simulink model "radix2_N128"  (R2024b)
settings: Solver=VariableStepAuto  StartTime=0.0  StopTime=1  RelTol=1e-3
settings Model: Creator=gjp88  LastModifiedBy=gjp88
settings SolverCC: AlgebraicLoopSolver=TrustRegion
settings DebuggingCC: UnconnectedInputMsg=warning  UnconnectedOutputMsg=warning  UnconnectedLineMsg=warning
settings ModelReferenceCC: EnableRefExpFcnMdlSchedulingChecks=on
settings RTWCC: GPUComputeCapability=3.5

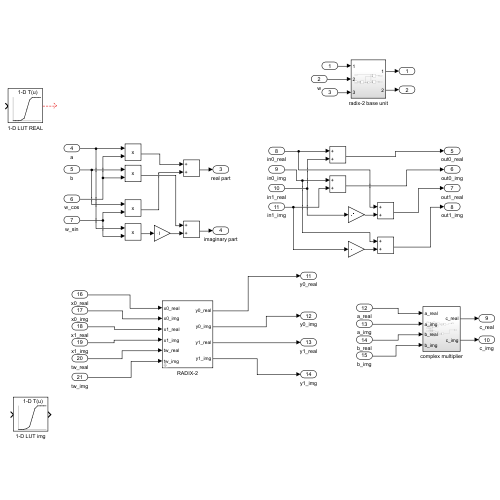
[thumbnail: Simulink's stored preview of the top-level diagram]
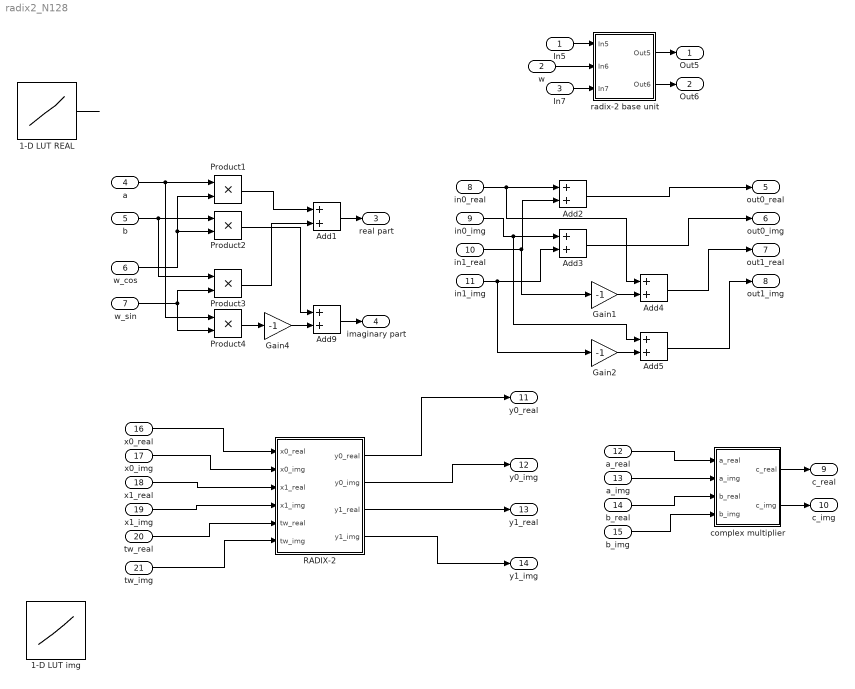
== system radix2_N128 ==
  In5 : Inport
  w : Inport  Port=2
  In7 : Inport  Port=3
  a : Inport  Port=4
  b : Inport  Port=5
  w_cos : Inport  Port=6
  w_sin : Inport  Port=7
  in0_real : Inport  Port=8
  in0_img : Inport  Port=9
  in1_real : Inport  Port=10
  in1_img : Inport  Port=11
  a_real : Inport  Port=12
  a_img : Inport  Port=13
  b_real : Inport  Port=14
  b_img : Inport  Port=15
  x0_real : Inport  Port=16
  x0_img : Inport  Port=17
  x1_real : Inport  Port=18
  x1_img : Inport  Port=19
  tw_real : Inport  Port=20
  tw_img : Inport  Port=21
  1-D LUT REAL : Lookup_n-D  NumberOfTableDimensions=1  BreakpointsForDimension1=[-5:5]  Table=tanh([-5:5])  InternalRulePriority=Speed  RndMeth=Simplest
  1-D LUT img : Lookup_n-D  NumberOfTableDimensions=1  BreakpointsForDimension1=[-5:5]  Table=tanh([-5:5])  InternalRulePriority=Speed  RndMeth=Simplest
  Add{1..5,9} (6 alike) : Sum
  Gain1 : Gain  Gain=-1
  Gain2 : Gain  Gain=-1
  Gain4 : Gain  Gain=-1
  Product{1..4} (4 alike) : Product
  RADIX-2 : Subsystem
      mask DialogControl RADIX_BUTTERFLY Prompt: RADIX-2
      mask DialogControl ParameterGroupVar Prompt: 参数
  complex multiplier : Subsystem
  radix-2 base unit : Subsystem
  Out5 : Outport
  Out6 : Outport  Port=2
  real part : Outport  Port=3
  imaginary part : Outport  Port=4
  out0_real : Outport  Port=5
  out0_img : Outport  Port=6
  out1_real : Outport  Port=7
  out1_img : Outport  Port=8
  c_real : Outport  Port=9
  c_img : Outport  Port=10
  y0_real : Outport  Port=11
  y0_img : Outport  Port=12
  y1_real : Outport  Port=13
  y1_img : Outport  Port=14
  wires:
  Gain4/1 -> Add9/2
  In5/1 -> radix-2 base unit/1(In5)
  a/1 -> Product4/1, Product1/1
  Product4/1 -> Gain4/1
  Add9/1 -> imaginary part/1
  Add1/1 -> real part/1
  Product1/1 -> Add1/1
  Product2/1 -> Add9/1
  Product3/1 -> Add1/2
  radix-2 base unit/2(Out6) -> Out6/1
  w_cos/1 -> Product2/2, Product1/2
  w/1 -> radix-2 base unit/2(In6)
  w_sin/1 -> Product3/2, Product4/2
  radix-2 base unit/1(Out5) -> Out5/1
  b/1 -> Product3/1, Product2/1
  In7/1 -> radix-2 base unit/3(In7)
  1-D LUT REAL/1 -> ?
  Gain1/1 -> Add4/2
  in0_real/1 -> Add4/1, Add2/1
  in1_real/1 -> Gain1/1, Add2/2
  Add4/1 -> out1_real/1
  Gain2/1 -> Add5/2
  in0_img/1 -> Add5/1, Add3/1
  in1_img/1 -> Gain2/1, Add3/2
  Add5/1 -> out1_img/1
  Add2/1 -> out0_real/1
  Add3/1 -> out0_img/1
  a_real/1 -> complex multiplier/1(a_real)
  a_img/1 -> complex multiplier/2(a_img)
  b_real/1 -> complex multiplier/3(b_real)
  b_img/1 -> complex multiplier/4(b_img)
  complex multiplier/1(c_real) -> c_real/1
  complex multiplier/2(c_img) -> c_img/1
  x0_real/1 -> RADIX-2/1(x0_real)
  x0_img/1 -> RADIX-2/2(x0_img)
  x1_real/1 -> RADIX-2/3(x1_real)
  x1_img/1 -> RADIX-2/4(x1_img)
  tw_real/1 -> RADIX-2/5(tw_real)
  tw_img/1 -> RADIX-2/6(tw_img)
  RADIX-2/1(y0_real) -> y0_real/1
  RADIX-2/2(y0_img) -> y0_img/1
  RADIX-2/3(y1_real) -> y1_real/1
  RADIX-2/4(y1_img) -> y1_img/1

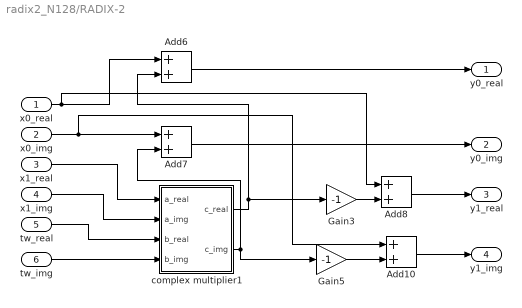
== system radix2_N128/RADIX-2 ==
  x0_real : Inport
  x0_img : Inport  Port=2
  x1_real : Inport  Port=3
  x1_img : Inport  Port=4
  tw_real : Inport  Port=5
  tw_img : Inport  Port=6
  Add{6..8,10} (4 alike) : Sum
  Gain3 : Gain  Gain=-1
  Gain5 : Gain  Gain=-1
  complex multiplier1 : Subsystem
  y0_real : Outport
  y0_img : Outport  Port=2
  y1_real : Outport  Port=3
  y1_img : Outport  Port=4
  wires:
  x0_img/1 -> Add10/1, Add7/1
  x1_real/1 -> complex multiplier1/1(a_real)
  Add10/1 -> y1_img/1
  tw_img/1 -> complex multiplier1/4(b_img)
  tw_real/1 -> complex multiplier1/3(b_real)
  Add7/1 -> y0_img/1
  Gain3/1 -> Add8/2
  x0_real/1 -> Add8/1, Add6/1
  Add6/1 -> y0_real/1
  complex multiplier1/2(c_img) -> Add7/2, Gain5/1
  Gain5/1 -> Add10/2
  complex multiplier1/1(c_real) -> Add6/2, Gain3/1
  x1_img/1 -> complex multiplier1/2(a_img)
  Add8/1 -> y1_real/1

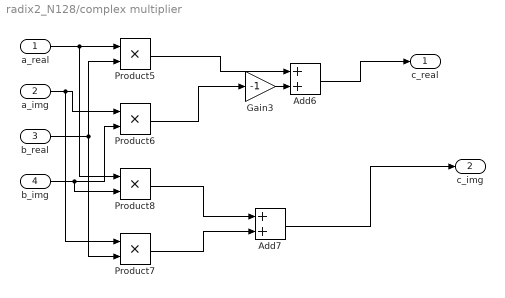
== system radix2_N128/complex multiplier ==
  a_real : Inport
  a_img : Inport  Port=2
  b_real : Inport  Port=3
  b_img : Inport  Port=4
  Add6 : Sum
  Add7 : Sum
  Gain3 : Gain  Gain=-1
  Product{5..8} (4 alike) : Product
  c_real : Outport
  c_img : Outport  Port=2
  wires:
  Product7/1 -> Add7/2
  Add6/1 -> c_real/1
  a_real/1 -> Product8/1, Product5/1
  Add7/1 -> c_img/1
  Product8/1 -> Add7/1
  Product5/1 -> Add6/1
  b_img/1 -> Product8/2, Product6/2
  a_img/1 -> Product7/1, Product6/1
  b_real/1 -> Product7/2, Product5/2
  Gain3/1 -> Add6/2
  Product6/1 -> Gain3/1

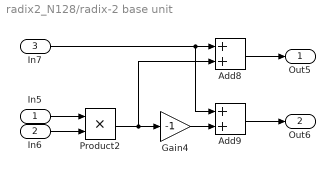
== system radix2_N128/radix-2 base unit ==
  In5 : Inport
  In6 : Inport  Port=2
  In7 : Inport  Port=3
  Add8 : Sum
  Add9 : Sum
  Gain4 : Gain  Gain=-1
  Product2 : Product
  Out5 : Outport
  Out6 : Outport  Port=2
  wires:
  In5/1 -> Product2/1
  In7/1 -> Add9/1, Add8/1
  Gain4/1 -> Add9/2
  Add8/1 -> Out5/1
  In6/1 -> Product2/2
  Add9/1 -> Out6/1
  Product2/1 -> Gain4/1, Add8/2

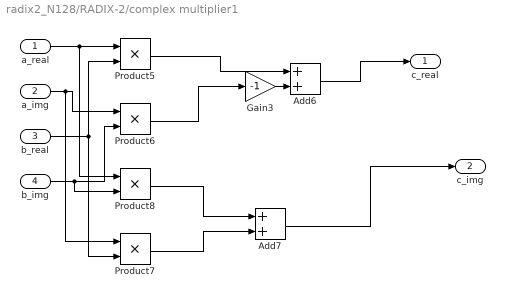
== system radix2_N128/RADIX-2/complex multiplier1 ==
  a_real : Inport
  a_img : Inport  Port=2
  b_real : Inport  Port=3
  b_img : Inport  Port=4
  Add6 : Sum
  Add7 : Sum
  Gain3 : Gain  Gain=-1
  Product{5..8} (4 alike) : Product
  c_real : Outport
  c_img : Outport  Port=2
  wires:
  Product7/1 -> Add7/2
  Add6/1 -> c_real/1
  a_real/1 -> Product8/1, Product5/1
  Add7/1 -> c_img/1
  Product8/1 -> Add7/1
  Product5/1 -> Add6/1
  b_img/1 -> Product8/2, Product6/2
  a_img/1 -> Product7/1, Product6/1
  b_real/1 -> Product7/2, Product5/2
  Gain3/1 -> Add6/2
  Product6/1 -> Gain3/1
